simulink model "test_main"  (R2018b)
settings: Solver=VariableStepAuto  StartTime=0.0  StopTime=600.0  RelTol=1e-3
libraries: CDH_command_lib x1, sgp4_lib_fsw x1, time_Lib x1
settings Model: Creator=Taylor  LastModifiedBy=Taylor

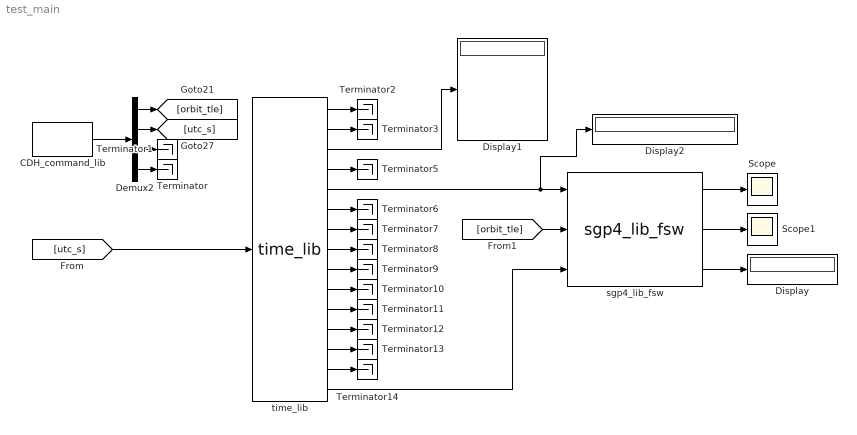
== system test_main ==
  CDH_command_lib : CDH_command_lib/CDH_command_lib  SystemSampleTime=-1
  Demux2 : Demux  Outputs=[9 1 3 7]
  Display : Display
  Display1 : Display
  Display2 : Display
  Scope : Scope
  Scope1 : Scope
  Terminator{,1..3,5..14} (14 alike) : Terminator
  sgp4_lib_fsw : sgp4_lib_fsw/sgp4_lib_fsw  SystemSampleTime=-1
  "time_lib " : time_Lib/time_lib    SystemSampleTime=-1
  wires:
  Demux2/3 -> Terminator1/1
  Demux2/2 -> [utc_s]
  Demux2/4 -> Terminator/1
  Demux2/1 -> [orbit_tle]
  CDH_command_lib/1 -> Demux2/1
  [utc_s] -> "time_lib "/1
  [orbit_tle] -> sgp4_lib_fsw/2
  "time_lib "/1 -> Terminator2/1
  "time_lib "/2 -> Terminator3/1
  "time_lib "/3 -> Display1/1
  "time_lib "/4 -> Terminator5/1
  "time_lib "/6 -> Terminator6/1
  "time_lib "/7 -> Terminator7/1
  "time_lib "/8 -> Terminator8/1
  "time_lib "/9 -> Terminator9/1
  "time_lib "/10 -> Terminator10/1
  "time_lib "/11 -> Terminator11/1
  "time_lib "/12 -> Terminator12/1
  "time_lib "/13 -> Terminator13/1
  "time_lib "/14 -> Terminator14/1
  sgp4_lib_fsw/1 -> Scope/1
  sgp4_lib_fsw/2 -> Scope1/1
  sgp4_lib_fsw/3 -> Display/1
  "time_lib "/5 -> Display2/1, sgp4_lib_fsw/1
  "time_lib "/15 -> sgp4_lib_fsw/3
